simulink model "L12AcutatorModel"  (R2014a)
settings: Solver=ode45  StartTime=StartTime  StopTime=StopTime  MaxStep=MaxStepSize  RelTol=1e-3
values from neighbouring files (symbols this model uses):
  K_backemf = min( K_backemf_array )    [ControlDesign.m]
  K_L12_Force = 2.29181    [ControlDesign.m]    (also in ControlDesignForceModeLinear.m)
  K_PWM = PWM_res/V_rail    (= 83.3333333333)    [ControlDesign.m]    (also in ControlDesignForceModeLinear.m = 0.012)
  Kspring = 55    [ControlDesign.m]    (also in ControlDesignForceModeLinear.m = 100)
  L12_Offset_I = 12.995    [ControlDesign.m]    (also in ControlDesignForceModeLinear.m)
  L_Range = [0 50]    [ControlDesign.m]    (also in ControlDesignForceModeLinear.m; VariableQpts.m)
  Mar = 0.075    [ControlDesign.m]    (also in ControlDesignForceModeLinear.m)
  Ra_L12 = 60    [ControlDesign.m]    (also in ControlDesignForceModeLinear.m)
settings Model: Creator=oberstare  LastModifiedBy=oberstar

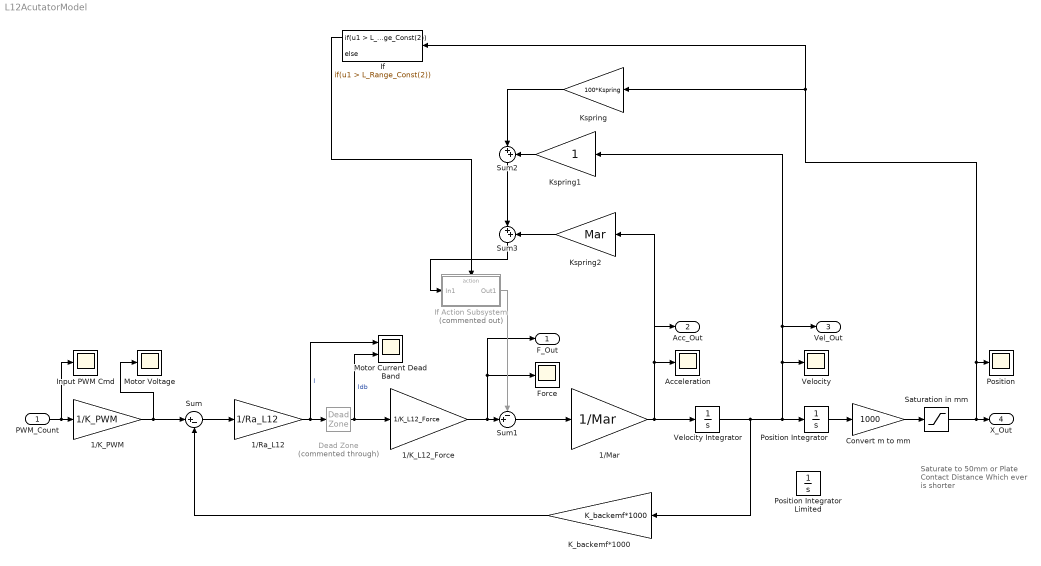
== system L12AcutatorModel ==
  note: Saturate to 50mm or
      | Plate Contact Distance
      | Which ever is shorter
  PWM_Count : Inport
  1/K_L12_Force : Gain  Gain=1/K_L12_Force
  1/K_PWM : Gain  Gain=1/K_PWM
  1/Mar : Gain  Gain=1/Mar
  1/Ra_L12 : Gain  Gain=1/Ra_L12
  Acceleration : Scope
      settings: YMin=-4.5  YMax=2  SaveName=ScopeData7
  Convert m to mm : Gain  Gain=1000
  Dead Zone : DeadZone  Commented=through  LowerValue=-L12_Offset_I/1000  UpperValue=L12_Offset_I/1000  SaturateOnIntegerOverflow=on
  Force : Scope
      settings: TimeRange=1  YMin=0.0795  YMax=0.084  SaveName=ScopeData8
  If : If  IfExpression=u1 > L_Range_Const(2)
  If Action Subsystem : Subsystem  Commented=on  TreatAsAtomicUnit=on
  Input PWM Cmd : Scope
      settings: AttributesFormatString=%<ShowName>  YMin=0  YMax=450  SaveName=ScopeData9
  K_backemf*1000 : Gain  Gain=K_backemf*1000
  Kspring : Gain  Gain=100*Kspring
  Kspring1 : Gain
  Kspring2 : Gain  Gain=Mar
  Motor Current Dead Band : Scope  NumInputPorts=2
      settings: YMin=0~0  YMax=0.35~0.325
  Motor Voltage : Scope
      settings: SaveName=ScopeData5
  Position : Scope
      settings: YMin=0  YMax=25  SaveName=ScopeData10
  Position Integrator : Integrator
  Position Integrator Limited : Integrator  LimitOutput=on  UpperSaturationLimit=50  LowerSaturationLimit=0
  Saturation in mm : Saturate  UpperLimit=L_Range(2)  LowerLimit=L_Range(1)
  Sum : Sum  Inputs=|+-
  Sum1 : Sum  Inputs=-+|
  Sum2 : Sum  Inputs=|++
  Sum3 : Sum  Inputs=|++
  Velocity : Scope
      settings: YMin=-0.005  YMax=0.007  SaveName=ScopeData11
  Velocity Integrator : Integrator
  F_Out : Outport
  Acc_Out : Outport  Port=2
  Vel_Out : Outport  Port=3
  X_Out : Outport  Port=4
  wires:
  PWM_Count/1 -> Input PWM Cmd/1, 1/K_PWM/1
  1/Mar/1 -> Kspring2/1, Acc_Out/1, Acceleration/1, Velocity Integrator/1
  Sum1/1 -> 1/Mar/1
  1/Ra_L12/1 -> Motor Current Dead Band/1, Dead Zone/1  "I"
  1/K_PWM/1 -> Sum/1, Motor Voltage/1
  Dead Zone/1 -> Motor Current Dead Band/2, 1/K_L12_Force/1  "Idb"
  Position Integrator/1 -> Convert m to mm/1
  Convert m to mm/1 -> Saturation in mm/1
  Sum/1 -> 1/Ra_L12/1
  K_backemf*1000/1 -> Sum/2
  1/K_L12_Force/1 -> Force/1, F_Out/1, Sum1/2
  Saturation in mm/1 -> Kspring/1, If/1, Position/1, X_Out/1
  Kspring/1 -> Sum2/1
  Kspring1/1 -> Sum2/2
  Velocity Integrator/1 -> Position Integrator/1, Kspring1/1, Vel_Out/1, Velocity/1, K_backemf*1000/1
  If Action Subsystem/1(Out1) -> Sum1/1
  If/1 -> If Action Subsystem/Action
  Sum2/1 -> Sum3/1
  Kspring2/1 -> Sum3/2
  Sum3/1 -> If Action Subsystem/1(In1)

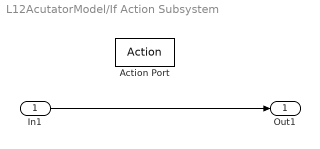
== system L12AcutatorModel/If Action Subsystem ==
  In1 : Inport
  Action Port : ActionPort  ActionType=then
  Out1 : Outport
  wires:
  In1/1 -> Out1/1
